simulink model "Subsystem"  (R2020b)
settings: Solver=VariableStepAuto  StartTime=0.0  StopTime=10.0  RelTol=1e-3
settings Model: Creator=WELCOME  LastModifiedBy=WELCOME
settings DataIOCC: SaveOutput=off  SaveTime=off

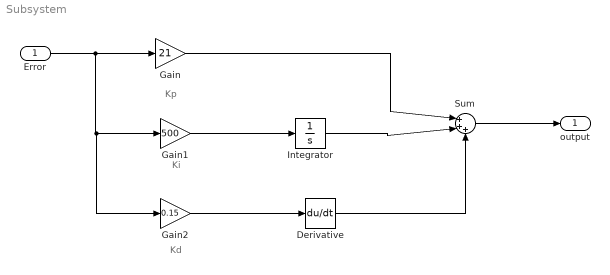
== system Subsystem ==
  note: Kd
  note: Ki
  note: Kp
  Error : Inport  OutDataTypeStr=double  PortDimensions=1  SampleTime=0
  Derivative : Derivative
  Gain : Gain  Gain=21
  Gain1 : Gain  Gain=500
  Gain2 : Gain  Gain=0.15
  Integrator : Integrator
  Sum : Sum  Inputs=|+++
  output : Outport  OutDataTypeStr=double  PortDimensions=1  SampleTime=0
  wires:
  Integrator/1 -> Sum/2
  Sum/1 -> output/1
  Error/1 -> Gain/1, Gain1/1, Gain2/1
  Derivative/1 -> Sum/3
  Gain1/1 -> Integrator/1
  Gain/1 -> Sum/1
  Gain2/1 -> Derivative/1
